simulink model "SiemensBike"  (R2025b)
settings: Solver=ode14x  StartTime=0  StopTime=inf  FixedStep=.01  RelTol=1e-2  EnableMultiTasking=on
StopFcn:
  | %toc
undefined symbols (not defined in the file): CtrlTcuInitGear, EnvAbsPrs, EnvAirTemp, EnvNomFrictionScaling, EnvNominalGrade, EnvWindVelX, EnvWindVelY, EnvWindVelZ, MotoFrmLngth, Sim3dSensor
libraries: vehdynlibviscommon x3, sim3dgroundtruthsensorlib x2, simulink x1, sharedtransform x1, autolibutils x1
(part 2 of 3)

== system SiemensBike/Environment/Friction/Varying Friction ==
  MotoFdbk : Inport
  Bus Selector1 : BusSelector  OutputSignals=Whl.Genrl.Frnt.Cp.Disp.x,Whl.Genrl.Rear.Cp.Disp.x,Whl.Genrl.Frnt.Cp.Disp.y,Whl.Genrl.Rear.Cp.Disp.y
  Bus Selector2 : BusSelector  OutputSignals=Body.InertFrm.Cg.Disp
  Road Track Friction : Subsystem  mask(Road Track Friction){surface_popup=Split friction coefficient scaling factor, lambda_g=EnvNomFrictionScaling, lambda_r=.6, r_x0=175, r_y0=-100, r_xw=1000, r_yw=500, aMode=2}
      mask prompts: surface_popup "vdynblks:vehdynManFriction:blkPrm_surface_popup"; lambda_g "vdynblks:vehdynManFriction:blkPrm_lambda_g"; lambda_r "vdynblks:vehdynManFriction:blkPrm_lambda_r"; r_x0 "vdynblks:vehdynManFriction:blkPrm_r_x0"; r_y0 "vdynblks:vehdynManFriction:blkPrm_r_y0"; r_xw "vdynblks:vehdynManFriction:blkPrm_r_xw"; r_yw "vdynblks:vehdynManFriction:blkPrm_r_yw"
      mask init:
      | % Scaling factor for the friction coefficient around the rectangular region
      | mutable = [lambda_g, lambda_g, lambda_g, lambda_g;
      |            lambda_g, lambda_r, lambda_r, lambda_g; 
      |            lambda_g, lambda_r, lambda_r, lambda_g; 
      |            lambda_g, lambda_g, lambda_g, lambda_g ];
      |        
      | 
      | % The step is distance between breakpoint near the boundary of high and
      | % low friction coefficient
      | 
      | step = 0.01 ; 
      | 
      | % In the mask initialization, xbr and ybr breakpoints are with respect to
      | % Body fixed coordinate system. At time t=0, xbr and ybr breakpoints
      | % updates to Earth (Inertial) Fixed coordinate system. The breakpoints for
      | % the lookup table are added via inputs.
      | 
      | xbr = [(r_x0 - step) , (r_x0 + step), (r_x0 + r_xw - step) , (r_x0 + r_xw + step) ];
      | ybr = [(r_y0 - step) , (r_y0 + step), (r_y0 + r_yw - step) , (r_y0 + r_yw + step) ];
      | 
      | 
      | % To check if the created track is split mu or constant mu
      | 
      | surface_popup = get_param(gcb, 'surface_popup');
      | 
      | if strcmp(surface_popup, 'Split friction coefficient scaling factor')
      |     SplitLambdaTrck = 1;
      | elseif strcmp(surface_popup, 'Constant friction coefficient scaling factor')
      |     SplitLambdaTrck = 0;
      | end
      mask Help: eval('vdynblkshelp(''vdynblkstrack'')');
      mask TypeOptions surface_popup: vdynblks:vehdynManFriction:blkCmb_surface_popup_c1 | vdynblks:vehdynManFriction:blkCmb_surface_popup_c2
      mask Callback surface_popup:
      | surface_popup = get_param(gcb, 'surface_popup');
      | m = Simulink.Mask.get(gcb);
      | 
      | lambda_g = m.getParameter('lambda_g');
      | lambda_r = m.getParameter('lambda_r');
      | r_x0 = m.getParameter('r_x0');
      | r_y0 = m.getParameter('r_y0');
      | r_xw = m.getParameter('r_xw');
      | r_yw = m.getParameter('r_yw');
      | %track_view = m.getParameter('track_view');
      | 
      | 
      | if strcmp(surface_popup, 'Split friction coefficient scaling factor')
      |     lambda_g.Visible = 'on';
      |     lambda_r.Visible = 'on';
      |     r_x0.Visible = 'on';
      |     r_y0.Visible = 'on';
      |     r_xw.Visible = 'on';
      |     r_yw.Visible = 'on';
      |     %track_view.Visible = 'on';
      | 
      | elseif strcmp(surface_popup,'Constant friction coefficient scaling factor')
      |     lambda_g.Visible = 'on';
      |     lambda_r.Visible = 'off';
      |     r_x0.Visible = 'off';
      |     r_y0.Visible = 'off';
      |     r_xw.Visible = 'off';
      |     r_yw.Visible = 'off';
      |     %track_view.Visible = 'off';
      | end
      | [~]=autosharedicon('autolibutils',gcb,0);
      mask DialogControl DescGroupVar Prompt: Road Track Friction
      mask DialogControl DescTextVar Prompt: vdynblks:vehdynManFriction:blkDesc
      mask DialogControl surface_popup Prompt: Type of surface:
      mask DialogControl lambda_g Prompt: Scaling factor for the friction coefficient of ground, lambda_g :
      mask DialogControl lambda_r Prompt: Scaling factor for the friction coefficient of rectangular surface, lambda_r :
      mask DialogControl r_x0 Prompt: X coordinate of lower left corner of rectangular surface, r_x0 [m]:
      mask DialogControl r_y0 Prompt: Y coordinate of lower left corner of rectangular surface, r_y0 [m]:
      mask DialogControl r_xw Prompt: Rectangular surface width in X direction, r_xw [m]:
      mask DialogControl r_yw Prompt: Rectangular surface width in Y direction, r_yw [m]:
  Wheel Coordinates : Subsystem
  FricCoeffLambda : Outport
  wires:
  Wheel Coordinates/1(XWhl) -> Road Track Friction/1(XWhl)
  MotoFdbk/1 -> Bus Selector2/1, Bus Selector1/1
  Wheel Coordinates/2(YWhl) -> Road Track Friction/2(YWhl)
  Road Track Friction/1(FricCoeffLambda) -> FricCoeffLambda/1
  Bus Selector2/1 -> Road Track Friction/3(Cg)  "<Disp>"
  Bus Selector1/1 -> Wheel Coordinates/1(FrntAxlX)  "<x>"
  Bus Selector1/2 -> Wheel Coordinates/2(RearAxlX)  "<x>"
  Bus Selector1/3 -> Wheel Coordinates/3(FrntAxlY)  "<y>"
  Bus Selector1/4 -> Wheel Coordinates/4(RearAxlY)  "<y>"

== system SiemensBike/Environment/Ground Feedback/3D Engine ==
  Friction : Inport
  WheelFdbk : Inport  Port=2
  3D Engine Source : Subsystem  Variant=on  VariantControl=Choice  mask(Terrain Source){terrType=Single point}
      mask prompts: terrType "Terrain feedback type:"
      mask help:
      | This variant subsystem provides the option for:
      | - a single point of contact for each wheel with minimal post-processing ideal for smooth surfaces and maximum run-time performance.
      | - multiple points of contact per wheel which may be used when interested in non-smooth terrain at a higher computational cost and requires Vehicle Dynamics Blockset.
      mask TypeOptions terrType: Single point | Multiple points
  Bus Creator2 : BusCreator  Inputs=2
  Bus Creator3 : BusCreator  Inputs=3
  Demux1 : Demux  Outputs=2
  Signal Specification1 : SignalSpecification  Unit=1
  Ground : Outport  VectorParamsAs1DForOutWhenUnconnected=off
  wires:
  3D Engine Source/2(DCM) -> Bus Creator3/2  "DCM"
  3D Engine Source/1(z) -> Bus Creator3/1  "z"
  WheelFdbk/1 -> 3D Engine Source/1(WheelFdbk)
  Friction/1 -> Signal Specification1/1
  Bus Creator3/1 -> Ground/1
  Bus Creator2/1 -> Bus Creator3/3  "mu"
  Demux1/2 -> Bus Creator2/2  "mu_R"
  Demux1/1 -> Bus Creator2/1  "mu_F"
  Signal Specification1/1 -> Demux1/1

== system SiemensBike/Environment/Ground Feedback/Constant ==
  Friction : Inport
  Bus Creator : BusCreator  Inputs=2
  Bus Creator2 : BusCreator  Inputs=2
  Bus Creator3 : BusCreator  Inputs=3
  Constant1 : Constant  Value=zeros(2,1)
  Constant2 : Constant  Value=repmat(eye(3),1,1,2)  SampleTime=-1
  Demux : Demux  Outputs=2
  Demux1 : Demux  Outputs=2
  Signal Specification : SignalSpecification  Unit=m
  Signal Specification1 : SignalSpecification  Unit=1
  Ground : Outport  VectorParamsAs1DForOutWhenUnconnected=off
  wires:
  Constant1/1 -> Signal Specification/1
  Signal Specification/1 -> Demux/1
  Demux/1 -> Bus Creator/1  "G_F_z"
  Demux/2 -> Bus Creator/2  "G_R_z"
  Bus Creator/1 -> Bus Creator3/1  "z"
  Demux1/1 -> Bus Creator2/1  "mu_F"
  Demux1/2 -> Bus Creator2/2  "mu_R"
  Bus Creator2/1 -> Bus Creator3/3  "mu"
  Friction/1 -> Signal Specification1/1
  Signal Specification1/1 -> Demux1/1
  Bus Creator3/1 -> Ground/1
  Constant2/1 -> Bus Creator3/2  "DCM"

== system SiemensBike/Motorcycle Vehicle/Body, Steer, Suspension, Wheels/Body, Steer, Suspension, Wheels ==
  WindXYZ : Inport
  BrkPrs : Inport  Port=2
  MDrvSprtR : Inport  Port=3
  MDrvArmR : Inport  Port=4
  MDrvFrm : Inport  Port=5
  ScaleFactrs : Inport  Port=6
  SteerCmd : Inport  Port=7
  In_Plane_Model : Subsystem  VariantControl=In_Plane_Model  ReferencedSubsystem=In_Plane_Model
  Out_of_Plane_Model : Subsystem  VariantControl=Out_of_Plane_Model  ReferencedSubsystem=Out_of_Plane_Model
  Moto : Outport
  Wheels : Outport  Port=2

== system SiemensBike/Motorcycle Vehicle/Body, Steer, Suspension, Wheels/Chassis Input ==
  Env : Inport
  Driveline : Inport  Port=2
  Rider : Inport  Port=3
  Bus Selector : BusSelector  OutputSignals=SteerFdbk
  Bus Selector2 : BusSelector  OutputSignals=Wind,Gnd.mu
  Bus Selector4 : BusSelector  OutputSignals=BrkPrs,Info.ChainInfo.MDrvSprtR,Info.MDrvArmR,Info.MDrvFrm
  Bus to Vector : BusToVector
  Wind : Outport  VectorParamsAs1DForOutWhenUnconnected=off
  BrkPrs : Outport  Port=2  VectorParamsAs1DForOutWhenUnconnected=off
  MDrvSprtR : Outport  Port=3  VectorParamsAs1DForOutWhenUnconnected=off
  MDrvArmR : Outport  Port=4  VectorParamsAs1DForOutWhenUnconnected=off
  MDrvFrm : Outport  Port=5  VectorParamsAs1DForOutWhenUnconnected=off
  ScaleFactrs : Outport  Port=6  VectorParamsAs1DForOutWhenUnconnected=off
  SteerCmd : Outport  Port=7  VectorParamsAs1DForOutWhenUnconnected=off
  wires:
  Env/1 -> Bus Selector2/1
  Bus Selector2/1 -> Wind/1  "<Wind>"
  Driveline/1 -> Bus Selector4/1
  Bus Selector4/4 -> MDrvFrm/1  "<MDrvFrm>"
  Bus Selector4/3 -> MDrvArmR/1  "<MDrvArmR>"
  Bus Selector4/2 -> MDrvSprtR/1  "<MDrvSprtR>"
  Bus Selector4/1 -> BrkPrs/1  "<BrkPrs>"
  Bus Selector2/2 -> Bus to Vector/1  "<mu>"
  Bus to Vector/1 -> ScaleFactrs/1
  Rider/1 -> Bus Selector/1
  Bus Selector/1 -> SteerCmd/1  "<SteerFdbk>"

== system SiemensBike/Motorcycle Vehicle/Body, Steer, Suspension, Wheels/Chassis Output ==
  Moto : Inport
  Wheels : Inport  Port=2
  Out Bus Element4 : Outport  PortName=MotoFdbk
  Out Bus Element1 : Outport  Port=2  PortName=WheelsFdbk
  wires:
  Moto/1 -> Out Bus Element4/1
  Wheels/1 -> Out Bus Element1/1

== system SiemensBike/Motorcycle Vehicle/Control Feedback/Variant Subsystem ==
  note: 1) Add Subsystem or Model blocks as valid variant choices.
      | 2) You cannot connect blocks at this level. At simulation, connectivity is automatically
      | determined, based on the active variant and port name matching.
  MotoFdbk : Inport
  IMU_Sensor : Subsystem  VariantControl=IMU_Sensor  ReferencedSubsystem=IMU_Sensor
  No_IMU_Sensor : Subsystem  VariantControl=No_IMU_Sensor  ReferencedSubsystem=No_IMU_Sensor
  IMU : Outport

== system SiemensBike/Motorcycle Vehicle/Hand Levers and Pedals/Hand Levers and Pedals ==
  note: Placeholder for introducing faults, detailed actuator behavior,
      | interactions of other systems with a human interface such
      | as changes in power steering and braking assistance.
  SteerCmd : Inport
  AccCmd : Inport  Port=2
  DecelCmd : Inport  Port=3
  GearCmd : Inport  Port=4
  BrkPrs : Inport  Port=5
  StrWhlTrq : Inport  Port=6
  Brake Pedal : Subsystem
  Dead Zone3 : DeadZone  LowerValue=-.01  UpperValue=.01  ZeroCross=off
  Terminator : Terminator
  Terminator1 : Terminator
  Twist2Acc : Lookup_n-D  NumberOfTableDimensions=1  BreakpointsForDimension1=[0 1]  Table=[0 1]  ExtrapMethod=Clip  InternalRulePriority=Speed  RndMeth=Simplest
  SteerFdbk : Outport
  AccFdbk : Outport  Port=2
  DecelFdbk : Outport  Port=3
  GearFdbk : Outport  Port=4
  wires:
  SteerCmd/1 -> Dead Zone3/1
  DecelCmd/1 -> Brake Pedal/1(DecelCmd)
  GearCmd/1 -> GearFdbk/1
  BrkPrs/1 -> Terminator/1
  StrWhlTrq/1 -> Terminator1/1
  Brake Pedal/1(DecelFdbk) -> DecelFdbk/1
  Dead Zone3/1 -> SteerFdbk/1
  AccCmd/1 -> Twist2Acc/1
  Twist2Acc/1 -> AccFdbk/1

== system SiemensBike/Motorcycle Vehicle/Hand Levers and Pedals/Pedal Cluster Input ==
  Rider : Inport
  Driveline : Inport  Port=2
  Bus Selector : BusSelector  OutputSignals=SteerCmd,AccelCmd,DecelCmd,GearCmd
  Bus Selector1 : BusSelector  OutputSignals=EMSpd
  Constant : Constant  Value=0
  SteerCmd : Outport  VectorParamsAs1DForOutWhenUnconnected=off
  AccelCmd : Outport  Port=2  VectorParamsAs1DForOutWhenUnconnected=off
  DecelCmd : Outport  Port=3  VectorParamsAs1DForOutWhenUnconnected=off
  GearCmd : Outport  Port=4  VectorParamsAs1DForOutWhenUnconnected=off
  BrkPrs : Outport  Port=5  VectorParamsAs1DForOutWhenUnconnected=off
  StrWhlTrq : Outport  Port=6  VectorParamsAs1DForOutWhenUnconnected=off
  wires:
  Bus Selector/2 -> AccelCmd/1  "<AccelCmd>"
  Rider/1 -> Bus Selector/1
  Bus Selector/3 -> DecelCmd/1  "<DecelCmd>"
  Bus Selector/4 -> GearCmd/1  "<GearCmd>"
  Bus Selector/1 -> SteerCmd/1  "<SteerCmd>"
  Driveline/1 -> Bus Selector1/1
  Bus Selector1/1 -> BrkPrs/1  "<EMSpd>"
  Constant/1 -> StrWhlTrq/1

== system SiemensBike/Motorcycle Vehicle/Hand Levers and Pedals/Pedal Cluster Output ==
  SteerFdbk : Inport
  AccFdbk : Inport  Port=2
  DecelFdbk : Inport  Port=3
  GearFdbk : Inport  Port=4
  Bus Creator1 : BusCreator  Inputs=4
  Signal Specification : SignalSpecification  Unit=N*m
  Signal Specification1 : SignalSpecification  Unit=1
  Signal Specification2 : SignalSpecification  Unit=1
  Signal Specification3 : SignalSpecification  Unit=1
  OperatorFdbk : Outport
  wires:
  Signal Specification1/1 -> Bus Creator1/2  "AccFdbk"
  Signal Specification3/1 -> Bus Creator1/4  "GearFdbk"
  AccFdbk/1 -> Signal Specification1/1
  DecelFdbk/1 -> Signal Specification2/1
  GearFdbk/1 -> Signal Specification3/1
  Signal Specification/1 -> Bus Creator1/1  "SteerFdbk"
  SteerFdbk/1 -> Signal Specification/1
  Bus Creator1/1 -> OperatorFdbk/1
  Signal Specification2/1 -> Bus Creator1/3  "DecelFdbk"

== system SiemensBike/Motorcycle Vehicle/Propulsion System/Actuators ==
  note: 1) Add Subsystem or Model blocks as valid variant choices.
      | 2) You cannot connect blocks at this level. At simulation, connectivity is automatically
      | determined, based on the active variant and port name matching.
  TrqCmd : Inport
  EngSpd : Inport  Port=2
  EMTrqCmd : Inport  Port=3
  EMSpd : Inport  Port=4
  AmbTemp : Inport  Port=5
  MotoElectricalSystem : Subsystem  VariantControl=MotoElectricalSystem  ReferencedSubsystem=MotoElectricalSystem
  MotoMappedEngine : Subsystem  VariantControl=MotoMappedEngine  ReferencedSubsystem=MotoMappedEngine
  MotoSimpleEngine : Subsystem  VariantControl=MotoSimpleEngine  ReferencedSubsystem=MotoSimpleEngine
  Eng : Outport
  Battery : Outport  Port=2
  ElecMachine : Outport  Port=3

== system SiemensBike/Motorcycle Vehicle/Propulsion System/Electrical System Input ==
  Cntrl : Inport
  Driveline : Inport  Port=2
  Env : Inport  Port=3
  Bus Selector : BusSelector  OutputSignals=VCU.EMTrqCmd
  Bus Selector1 : BusSelector  OutputSignals=EMSpd
  Bus Selector2 : BusSelector  OutputSignals=Temp
  First Order Hold : FirstOrderHold  ErrorTolerance=inf  AllowContinuousInput=on
  EMTrqCmd : Outport  VectorParamsAs1DForOutWhenUnconnected=off
  EMSpd : Outport  Port=2  VectorParamsAs1DForOutWhenUnconnected=off
  AmbTemp : Outport  Port=3  VectorParamsAs1DForOutWhenUnconnected=off
  wires:
  Cntrl/1 -> Bus Selector/1
  Bus Selector/1 -> First Order Hold/1  "<EMTrqCmd>"
  Bus Selector1/1 -> EMSpd/1  "<EMSpd>"
  Env/1 -> Bus Selector2/1
  Bus Selector2/1 -> AmbTemp/1  "<Temp>"
  Driveline/1 -> Bus Selector1/1
  First Order Hold/1 -> EMTrqCmd/1

== system SiemensBike/Motorcycle Vehicle/Propulsion System/Engine Input ==
  Cntrl : Inport
  Driveline : Inport  Port=2
  Bus Selector : BusSelector  OutputSignals=ECU.EngTrqCmd
  Bus Selector1 : BusSelector  OutputSignals=EngSpd
  First Order Hold : FirstOrderHold  OutputAlgorithm=Fast (Minimize Error)  ErrorTolerance=.01  AllowContinuousInput=on
  EngTrqCmd : Outport  VectorParamsAs1DForOutWhenUnconnected=off
  EngSpd : Outport  Port=2  VectorParamsAs1DForOutWhenUnconnected=off
  wires:
  Driveline/1 -> Bus Selector1/1
  Cntrl/1 -> Bus Selector/1
  Bus Selector/1 -> First Order Hold/1  "<EngTrqCmd>"
  Bus Selector1/1 -> EngSpd/1  "<EngSpd>"
  First Order Hold/1 -> EngTrqCmd/1

== system SiemensBike/Motorcycle Vehicle/Transmission, Driveline and Brakes/Brake Hydraulics ==
  BrkPrsCmd : Inport
  Front Bias : Constant
  Gain4 : Gain  Gain=8e6
  Mux : Mux  Inputs=2
  Product : Product
  Rear Bias : Constant  Value=.6
  Valve : autolibutils/Cont LPF  wc=20*2*pi  AbsoluteTolerance=auto  aMode=2
  BrkPrs : Outport  VectorParamsAs1DForOutWhenUnconnected=off
  wires:
  Valve/1 -> Product/2
  Gain4/1 -> BrkPrs/1
  BrkPrsCmd/1 -> Valve/1
  Front Bias/1 -> Mux/1
  Rear Bias/1 -> Mux/2
  Product/1 -> Gain4/1
  Mux/1 -> Product/1

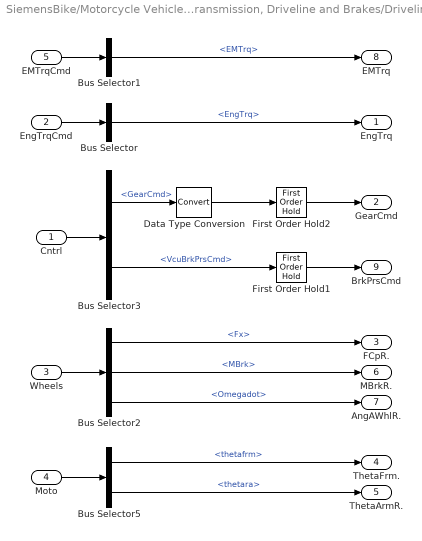
== system SiemensBike/Motorcycle Vehicle/Transmission, Driveline and Brakes/Driveline Input ==
  Cntrl : Inport
  EngTrqCmd : Inport  Port=2
  Wheels : Inport  Port=3
  Moto : Inport  Port=4
  EMTrqCmd : Inport  Port=5
  Bus Selector : BusSelector  OutputSignals=EngTrq
  Bus Selector1 : BusSelector  OutputSignals=EMTrq
  Bus Selector2 : BusSelector  OutputSignals=RearTire.Fx,RearTire.MBrk,RearTire.Omegadot
  Bus Selector3 : BusSelector  OutputSignals=Transmission.GearCmd,VCU.VcuBrkPrsCmd
  Bus Selector5 : BusSelector  OutputSignals=Frame.Genrl.Ang.thetafrm,RearArm.Genrl.Ang.thetara
  Data Type Conversion : DataTypeConversion  SaturateOnIntegerOverflow=off  RndMeth=Floor
  First Order Hold1 : FirstOrderHold  OutputAlgorithm=Fast (Minimize Error)  ErrorTolerance=.001  AllowContinuousInput=on
  First Order Hold2 : FirstOrderHold  InitialOutput=CtrlTcuInitGear  ErrorTolerance=.5  AllowContinuousInput=on
  EngTrq : Outport  VectorParamsAs1DForOutWhenUnconnected=off
  GearCmd : Outport  Port=2  VectorParamsAs1DForOutWhenUnconnected=off
  FCpR. : Outport  Port=3  VectorParamsAs1DForOutWhenUnconnected=off
  ThetaFrm. : Outport  Port=4  VectorParamsAs1DForOutWhenUnconnected=off
  ThetaArmR. : Outport  Port=5  VectorParamsAs1DForOutWhenUnconnected=off
  MBrkR. : Outport  Port=6  VectorParamsAs1DForOutWhenUnconnected=off
  AngAWhlR. : Outport  Port=7  VectorParamsAs1DForOutWhenUnconnected=off
  EMTrq : Outport  Port=8  VectorParamsAs1DForOutWhenUnconnected=off
  BrkPrsCmd : Outport  Port=9  VectorParamsAs1DForOutWhenUnconnected=off
  wires:
  Wheels/1 -> Bus Selector2/1
  Moto/1 -> Bus Selector5/1
  Bus Selector2/3 -> AngAWhlR./1  "<Omegadot>"
  Bus Selector2/2 -> MBrkR./1  "<MBrk>"
  Bus Selector2/1 -> FCpR./1  "<Fx>"
  Bus Selector5/2 -> ThetaArmR./1  "<thetara>"
  Bus Selector5/1 -> ThetaFrm./1  "<thetafrm>"
  EngTrqCmd/1 -> Bus Selector/1
  EMTrqCmd/1 -> Bus Selector1/1
  Bus Selector3/2 -> First Order Hold1/1  "<VcuBrkPrsCmd>"
  Bus Selector3/1 -> Data Type Conversion/1  "<GearCmd>"
  Cntrl/1 -> Bus Selector3/1
  Bus Selector/1 -> EngTrq/1  "<EngTrq>"
  Bus Selector1/1 -> EMTrq/1  "<EMTrq>"
  First Order Hold1/1 -> BrkPrsCmd/1
  Data Type Conversion/1 -> First Order Hold2/1
  First Order Hold2/1 -> GearCmd/1

== system SiemensBike/Motorcycle Vehicle/Transmission, Driveline and Brakes/Driveline Output ==
  EngSpd : Inport
  Gear : Inport  Port=2
  Info : Inport  Port=3
  EMSpd : Inport  Port=4
  BrkPrs : Inport  Port=5
  Bus Creator1 : BusCreator  Inputs=7
  Ground{,1..3} (4 alike) : Ground
  Mux : Mux  Inputs=2
  Mux1 : Mux  Inputs=2
  Signal Specification7 : SignalSpecification  Unit=Pa  Dimensions=2
  Driveline : Outport  VectorParamsAs1DForOutWhenUnconnected=off
  wires:
  Bus Creator1/1 -> Driveline/1  "Driveline"
  EngSpd/1 -> Bus Creator1/3  "EngSpd"
  EMSpd/1 -> Bus Creator1/2  "EMSpd"
  Gear/1 -> Bus Creator1/4  "Gear"
  Info/1 -> Bus Creator1/7  "Info"
  Mux/1 -> Bus Creator1/6  "AxlTrq"
  Mux1/1 -> Bus Creator1/5  "PropShftSpd"
  Ground3/1 -> Mux/2
  Ground2/1 -> Mux/1
  Ground/1 -> Mux1/1
  Ground1/1 -> Mux1/2
  BrkPrs/1 -> Signal Specification7/1
  Signal Specification7/1 -> Bus Creator1/1  "BrkPrs"

== system SiemensBike/Motorcycle Vehicle/Transmission, Driveline and Brakes/Transmission and Driveline ==
  EngTrq : Inport
  GearCmd : Inport  Port=2
  FCpR : Inport  Port=3
  ThetaFrm : Inport  Port=4
  ThetaArmR : Inport  Port=5
  MBrkR : Inport  Port=6
  AngAWhlR : Inport  Port=7
  EMTrq : Inport  Port=8
  Driveline : Subsystem  Variant=on  VariantChoicesSpecifier={'Chain_Drive', 'No_Chain_Drive'}  VariantControlMode=label  VariantControl=Choice  LabelModeActiveChoice=Chain_Drive
  Transmission : Subsystem  Variant=on  VariantChoicesSpecifier={'ConventionalMotorcycle', 'ElectricMotorcycle'}  VariantControlMode=label  VariantControl=Choice  LabelModeActiveChoice=ConventionalMotorcycle
  EngSpd : Outport
  Gear : Outport  Port=2
  Info : Outport  Port=3
  EMSpd : Outport  Port=4
  wires:
  EngTrq/1 -> Transmission/1(EngTrq)
  GearCmd/1 -> Transmission/2(GearCmd)
  FCpR/1 -> Driveline/1(FCpR)
  ThetaFrm/1 -> Driveline/2(ThetaFrm)
  ThetaArmR/1 -> Driveline/3(ThetaArmR)
  MBrkR/1 -> Driveline/4(MBrkR)
  AngAWhlR/1 -> Driveline/5(AngAWhlR)
  EMTrq/1 -> Transmission/3(EMTrq)
  Driveline/2(DrvSprktSpd) -> Transmission/4(DrvSprktSpd)
  Transmission/4(DrvSprktTrq) -> Driveline/6(DrvSprktTrq)
  Driveline/1(Info) -> Info/1
  Transmission/1(EngSpd) -> EngSpd/1
  Transmission/2(Gear) -> Gear/1
  Transmission/3(EMSpd) -> EMSpd/1

== system SiemensBike/Visualization/ISO 15037-1:2006/Disabled ==
  VehFdbk : Inport
  Terminator1 : Terminator
  wires:
  VehFdbk/1 -> Terminator1/1

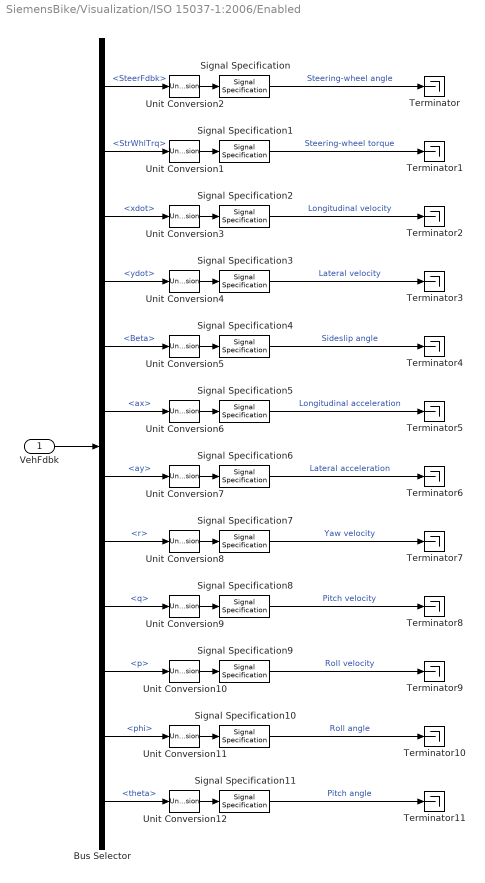
== system SiemensBike/Visualization/ISO 15037-1:2006/Enabled ==
  VehFdbk : Inport
  Bus Selector : BusSelector  OutputSignals=Rider.SteerFdbk,Steering.StrWhlTrq,Body.BdyFrm.Cg.Vel.xdot,Body.BdyFrm.Cg.Vel.ydot,Body.BdyFrm.Cg.Ang.Beta,Body.BdyFrm.Cg.Acc.ax,Body.BdyFrm.Cg.Acc.ay,Body.BdyFrm.Cg.AngVel.r,Body.BdyFrm.Cg.AngVel.q,Body.BdyFrm.Cg.AngVel.p,Body.InertFrm.Cg.Ang.phi,Body.InertFrm.Cg.Ang.theta
  Signal Specification{,4,10..11} (4 alike) : SignalSpecification  Unit=deg
  Signal Specification1 : SignalSpecification  Unit=N*m
  Signal Specification2 : SignalSpecification  Unit=km/h
  Signal Specification3 : SignalSpecification  Unit=m/s
  Signal Specification5 : SignalSpecification  Unit=m/s^2
  Signal Specification6 : SignalSpecification  Unit=m/s^2
  Signal Specification7 : SignalSpecification  Unit=deg/s
  Signal Specification8 : SignalSpecification  Unit=deg/s
  Signal Specification9 : SignalSpecification  Unit=deg/s
  Terminator{,1..11} (12 alike) : Terminator
  Unit Conversion{1..12} (12 alike) : UnitConversion
  wires:
  Bus Selector/12 -> Unit Conversion12/1  "<theta>"
  Signal Specification11/1 -> Terminator11/1  "Pitch angle"
  Unit Conversion12/1 -> Signal Specification11/1
  Bus Selector/11 -> Unit Conversion11/1  "<phi>"
  Unit Conversion11/1 -> Signal Specification10/1
  Signal Specification10/1 -> Terminator10/1  "Roll angle"
  Bus Selector/10 -> Unit Conversion10/1  "<p>"
  Signal Specification9/1 -> Terminator9/1  "Roll velocity"
  Unit Conversion10/1 -> Signal Specification9/1
  Bus Selector/9 -> Unit Conversion9/1  "<q>"
  Unit Conversion9/1 -> Signal Specification8/1
  Signal Specification8/1 -> Terminator8/1  "Pitch velocity"
  Bus Selector/8 -> Unit Conversion8/1  "<r>"
  Signal Specification7/1 -> Terminator7/1  "Yaw velocity"
  Unit Conversion8/1 -> Signal Specification7/1
  Bus Selector/7 -> Unit Conversion7/1  "<ay>"
  Unit Conversion7/1 -> Signal Specification6/1
  Signal Specification6/1 -> Terminator6/1  "Lateral acceleration"
  Bus Selector/6 -> Unit Conversion6/1  "<ax>"
  Signal Specification5/1 -> Terminator5/1  "Longitudinal acceleration"
  Unit Conversion6/1 -> Signal Specification5/1
  Bus Selector/5 -> Unit Conversion5/1  "<Beta>"
  Unit Conversion5/1 -> Signal Specification4/1
  Signal Specification4/1 -> Terminator4/1  "Sideslip angle"
  Bus Selector/4 -> Unit Conversion4/1  "<ydot>"
  Signal Specification3/1 -> Terminator3/1  "Lateral velocity"
  Unit Conversion4/1 -> Signal Specification3/1
  Bus Selector/3 -> Unit Conversion3/1  "<xdot>"
  Unit Conversion3/1 -> Signal Specification2/1
  Signal Specification2/1 -> Terminator2/1  "Longitudinal velocity"
  Signal Specification1/1 -> Terminator1/1  "Steering-wheel torque"
  Unit Conversion1/1 -> Signal Specification1/1
  Bus Selector/2 -> Unit Conversion1/1  "<StrWhlTrq>"
  Signal Specification/1 -> Terminator/1  "Steering-wheel angle"
  Unit Conversion2/1 -> Signal Specification/1
  VehFdbk/1 -> Bus Selector/1
  Bus Selector/1 -> Unit Conversion2/1  "<SteerFdbk>"

== system SiemensBike/Visualization/Scope Type/DLC ==
  VehFdbk : Inport
  Vis : Inport  Port=2
  Bus Creator : BusCreator  Inputs=3
  Bus Selector3 : BusSelector  OutputSignals=Body.InertFrm.Cg.Disp.X,Body.InertFrm.Cg.Disp.Z
  Bus Selector4 : BusSelector  OutputSignals=LeftBnd,RightBnd,LtrlRef
  Lane Change : Scope
      settings: Title=Double Lane Change: Lateral Displacement  ActiveDisplayYMinimum=-3.28469  ActiveDisplayYMaximum=6.06905  YLabel=Lateral Displacement [m] (positive = right direction)  DataLoggingSaveFormat=Array
  Mux1 : Mux  Inputs=3
  Rate Transition : RateTransition  OutPortSampleTime=.1
  Rate Transition3 : RateTransition  OutPortSampleTime=.1
  Signal Copy : SignalConversion  OverrideOpt=off
  Signal Copy1 : SignalConversion  OverrideOpt=off
  Signal Copy2 : SignalConversion  OverrideOpt=off
  Ref : Outport  VectorParamsAs1DForOutWhenUnconnected=off
  wires:
  VehFdbk/1 -> Bus Selector3/1
  Vis/1 -> Bus Selector4/1
  Bus Creator/1 -> Ref/1
  Bus Selector3/2 -> Signal Copy2/1  "<Z>"
  Signal Copy/1 -> Bus Creator/2  "YRef"
  Signal Copy1/1 -> Bus Creator/1  "XRef"
  Signal Copy2/1 -> Bus Creator/3  "ZRef"
  Rate Transition3/1 -> Mux1/2  "Right Boundary"
  Bus Selector4/3 -> Signal Copy/1, Mux1/3  "<LtrlRef>"
  Mux1/1 -> Lane Change/1
  Bus Selector4/1 -> Rate Transition/1  "<LeftBnd>"
  Rate Transition/1 -> Mux1/1  "Left Boundary"
  Bus Selector4/2 -> Rate Transition3/1  "<RightBnd>"
  Bus Selector3/1 -> Signal Copy1/1  "<X>"

== system SiemensBike/Visualization/Scope Type/None ==
  VehFdbk : Inport
  Vis : Inport  Port=2
  Bus Selector2 : BusSelector  OutputSignals=Steer.Genrl.Ang.thetasteer
  Bus Selector9 : BusSelector  OutputSignals=Body.BdyFrm.Cg.AngVel.r
  Signal Specification3 : SignalSpecification  Unit=deg/s
  Unit Conversion4 : UnitConversion
  Yaw Rate and Steer : Scope  NumInputPorts=2
      settings: ActiveDisplayYMinimum=-112.49987  ActiveDisplayYMaximum=112.49996
  Ref : Outport  VectorParamsAs1DForOutWhenUnconnected=off
  wires:
  Bus Selector9/1 -> Unit Conversion4/1  "<r>"
  Signal Specification3/1 -> Yaw Rate and Steer/1
  Unit Conversion4/1 -> Signal Specification3/1
  VehFdbk/1 -> Bus Selector2/1, Bus Selector9/1  "VehFdbk"
  Bus Selector2/1 -> Yaw Rate and Steer/2  "<thetasteer>"
  Vis/1 -> Ref/1

== system SiemensBike/Visualization/Scope Type/XYZ ==
  VehFdbk : Inport
  Vis : Inport  Port=2
  Terminator : Terminator
  Ref : Outport  VectorParamsAs1DForOutWhenUnconnected=off
  wires:
  Vis/1 -> Ref/1
  VehFdbk/1 -> Terminator/1

== system SiemensBike/Visualization/Vehicle XY Plotter/Disabled ==

== system SiemensBike/Visualization/Vehicle XY Plotter/XY View ==
  Bus Element In2 : Inport  PortName=VehFdbk
  Bus Selector1 : BusSelector  OutputSignals=Body.InertFrm.Cg.Ang.phi,Body.InertFrm.Cg.Ang.theta,Body.InertFrm.Cg.Ang.psi  OutputAsBus=on
  Bus Selector2 : BusSelector  OutputSignals=Wheels.FrontTire.Fx,Wheels.RearTire.Fx
  Bus Selector3 : BusSelector  OutputSignals=Wheels.FrontTire.Fy,Wheels.RearTire.Fy
  Bus Selector5 : BusSelector  OutputSignals=Wheels.FrontTire.Alpha,Wheels.RearTire.Alpha
  Bus Selector6 : BusSelector  OutputSignals=Body.InertFrm.Cg.Disp.X,Body.InertFrm.Cg.Disp.Y,Body.InertFrm.Cg.Disp.Z  OutputAsBus=on
  Bus Selector7 : BusSelector  OutputSignals=Body.InertFrm.Cg.Vel.Xdot,Body.InertFrm.Cg.Vel.Ydot,Body.InertFrm.Cg.Vel.Zdot  OutputAsBus=on
  Bus Selector9 : BusSelector  OutputSignals=Driveline.EngSpd,Driveline.EMSpd,Driveline.Gear
  Bus to Vector : BusToVector
  Bus to Vector1 : BusToVector
  Bus to Vector2 : BusToVector
  Max : MinMax  Function=max  Inputs=2
  Multi-Track XY Plotter : vehdynlibviscommon/Multi-Track XY Plotter  numTrack=Single track  extRef=off  extStats=on  extTireF=on  a=1.5  b=1.5  w=0  figBorder=10  bufferSize=1024  velNorm=5  tireFNorm=1000  pltDT=.1
      settings: LibrarySourceBlock=vehdynlibviscommon/Vehicle XY Plot Configuration
  Mux{,1..3} (4 alike) : Mux  Inputs=2
  Unary Minus : UnaryMinus
  wires:
  Bus Selector7/1 -> Bus to Vector1/1
  Bus to Vector1/1 -> Multi-Track XY Plotter/3
  Bus Selector2/1 -> Mux1/1  "<Fx>"
  Bus Selector1/1 -> Bus to Vector2/1
  Bus Selector9/1 -> Max/1  "<EngSpd>"
  Bus to Vector/1 -> Multi-Track XY Plotter/1
  Bus Selector6/1 -> Bus to Vector/1
  Bus to Vector2/1 -> Multi-Track XY Plotter/2
  Bus Element In2/1 -> Bus Selector3/1, Bus Selector2/1, Bus Selector9/1, Bus Selector5/1, Bus Selector7/1, Bus Selector1/1, Bus Selector6/1  "VehFdbk"
  Mux3/1 -> Multi-Track XY Plotter/4
  Mux1/1 -> Multi-Track XY Plotter/6
  Mux2/1 -> Unary Minus/1
  Max/1 -> Mux/1
  Bus Selector9/2 -> Max/2  "<EMSpd>"
  Mux/1 -> Multi-Track XY Plotter/5
  Bus Selector9/3 -> Mux/2  "<Gear>"
  Bus Selector2/2 -> Mux1/2  "<Fx>"
  Bus Selector3/2 -> Mux2/2  "<Fy>"
  Bus Selector3/1 -> Mux2/1  "<Fy>"
  Bus Selector5/1 -> Mux3/1  "<Alpha>"
  Bus Selector5/2 -> Mux3/2  "<Alpha>"
  Unary Minus/1 -> Multi-Track XY Plotter/7

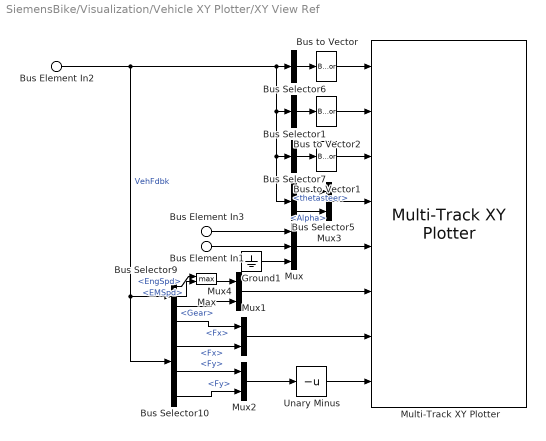
== system SiemensBike/Visualization/Vehicle XY Plotter/XY View Ref ==
  Bus Element In2 : Inport  PortName=VehFdbk
  Bus Element In1 : Inport  Port=2  PortName=Ref  Element=YRef
  Bus Element In3 : Inport  Port=2  PortName=Ref  Element=XRef
  Bus Selector1 : BusSelector  OutputSignals=Body.InertFrm.Cg.Ang.phi,Body.InertFrm.Cg.Ang.theta,Body.InertFrm.Cg.Ang.psi  OutputAsBus=on
  Bus Selector10 : BusSelector  OutputSignals=Wheels.FrontTire.Fx,Wheels.RearTire.Fx,Wheels.FrontTire.Fy,Wheels.RearTire.Fy
  Bus Selector5 : BusSelector  OutputSignals=Steer.Genrl.Ang.thetasteer,Wheels.RearTire.Alpha
  Bus Selector6 : BusSelector  OutputSignals=Body.InertFrm.Cg.Disp.X,Body.InertFrm.Cg.Disp.Y,Body.InertFrm.Cg.Disp.Z  OutputAsBus=on
  Bus Selector7 : BusSelector  OutputSignals=Body.InertFrm.Cg.Vel.Xdot,Body.InertFrm.Cg.Vel.Ydot,Body.InertFrm.Cg.Vel.Zdot  OutputAsBus=on
  Bus Selector9 : BusSelector  OutputSignals=Driveline.EngSpd,Driveline.EMSpd,Driveline.Gear
  Bus to Vector : BusToVector
  Bus to Vector1 : BusToVector
  Bus to Vector2 : BusToVector
  Ground1 : Ground
  Max : MinMax  Function=max  Inputs=2
  Multi-Track XY Plotter : vehdynlibviscommon/Multi-Track XY Plotter  numTrack=Single track  extRef=on  extStats=on  extTireF=on  a=1.5  b=1.5  w=0  figBorder=10  bufferSize=1024  velNorm=5  tireFNorm=1000  pltDT=.1
      settings: LibrarySourceBlock=vehdynlibviscommon/Vehicle XY Plot Configuration
  Mux : Mux  Inputs=3
  Mux{1..4} (4 alike) : Mux  Inputs=2
  Unary Minus : UnaryMinus
  wires:
  Bus Selector7/1 -> Bus to Vector1/1
  Ground1/1 -> Mux/3
  Mux2/1 -> Unary Minus/1
  Bus to Vector1/1 -> Multi-Track XY Plotter/3
  Mux1/1 -> Multi-Track XY Plotter/7
  Bus Selector1/1 -> Bus to Vector2/1
  Bus Element In1/1 -> Mux/2
  Mux4/1 -> Multi-Track XY Plotter/6
  Bus Element In3/1 -> Mux/1
  Mux/1 -> Multi-Track XY Plotter/5
  Bus to Vector/1 -> Multi-Track XY Plotter/1
  Bus Selector6/1 -> Bus to Vector/1
  Bus to Vector2/1 -> Multi-Track XY Plotter/2
  Bus Selector5/1 -> Mux3/1  "<thetasteer>"
  Mux3/1 -> Multi-Track XY Plotter/4
  Bus Selector5/2 -> Mux3/2  "<Alpha>"
  Bus Selector10/1 -> Mux1/1  "<Fx>"
  Bus Selector10/2 -> Mux1/2  "<Fx>"
  Bus Selector10/3 -> Mux2/1  "<Fy>"
  Bus Selector10/4 -> Mux2/2  "<Fy>"
  Unary Minus/1 -> Multi-Track XY Plotter/8
  Bus Selector9/3 -> Mux4/2  "<Gear>"
  Bus Selector9/1 -> Max/1  "<EngSpd>"
  Bus Selector9/2 -> Max/2  "<EMSpd>"
  Max/1 -> Mux4/1
  Bus Element In2/1 -> Bus Selector9/1, Bus Selector10/1, Bus Selector5/1, Bus Selector7/1, Bus Selector1/1, Bus Selector6/1  "VehFdbk"

== system SiemensBike/Environment/Friction/Varying Friction/Road Track Friction ==
  XWhl : Inport
  YWhl : Inport  Port=2
  Cg : Inport  Port=3
  2D Lookup Tbl for Scaling Fctr (Lambda) : Subsystem  TreatAsAtomicUnit=on
      mask init:
      | [~]=vehdynicon('vehdynblk',gcb);
  Bus Selector : BusSelector  OutputSignals=X,Y
  Cnst Lambda : Constant  Value=ones(2,1).*lambda_g
  Constant1 : Constant  Value=SplitLambdaTrck
  Creating Inertial Frm Bpt : Subsystem
  En at t = 0 : Subsystem
  "Lambda (t = 0) " : Memory  InitialCondition=ones(2,1).*lambda_g  InheritSampleTime=on
  Switch : Switch  Criteria=u2 > Threshold  ZeroCross=off  SaturateOnIntegerOverflow=off  InputSameDT=off
  FricCoeffLambda : Outport
  wires:
  YWhl/1 -> 2D Lookup Tbl for Scaling Fctr (Lambda)/2(YWhl)
  XWhl/1 -> 2D Lookup Tbl for Scaling Fctr (Lambda)/1(XWhl)
  2D Lookup Tbl for Scaling Fctr (Lambda)/1(Lambda for each whl) -> Switch/1
  "Lambda (t = 0) "/1 -> FricCoeffLambda/1
  Switch/1 -> "Lambda (t = 0) "/1
  Cnst Lambda/1 -> Switch/3
  Constant1/1 -> Switch/2
  Cg/1 -> Bus Selector/1
  Creating Inertial Frm Bpt/1(XBpt) -> 2D Lookup Tbl for Scaling Fctr (Lambda)/3(XBpt)
  Creating Inertial Frm Bpt/2(YBpt) -> 2D Lookup Tbl for Scaling Fctr (Lambda)/4(YBpt)
  Bus Selector/1 -> Creating Inertial Frm Bpt/1(XCg)  "<X>"
  Bus Selector/2 -> Creating Inertial Frm Bpt/2(YCg)  "<Y>"
  En at t = 0/1(Out1) -> Creating Inertial Frm Bpt/Enable

== system SiemensBike/Environment/Friction/Varying Friction/Wheel Coordinates ==
  FrntAxlX : Inport
  RearAxlX : Inport  Port=2
  FrntAxlY : Inport  Port=3
  RearAxlY : Inport  Port=4
  Matrix Concatenate : Concatenate  Mode=Multidimensional array
  Matrix Concatenate1 : Concatenate  Mode=Multidimensional array
  XWhl : Outport
  YWhl : Outport  Port=2
  wires:
  Matrix Concatenate/1 -> XWhl/1
  FrntAxlX/1 -> Matrix Concatenate/1
  Matrix Concatenate1/1 -> YWhl/1
  FrntAxlY/1 -> Matrix Concatenate1/1
  RearAxlY/1 -> Matrix Concatenate1/2
  RearAxlX/1 -> Matrix Concatenate/2

== system SiemensBike/Environment/Ground Feedback/3D Engine/3D Engine Source ==
  WheelFdbk : Inport
  Multiple Points : Subsystem  VariantControl=terrType==2
  Single Point : Subsystem  VariantControl=terrType ==1
  z : Outport
  DCM : Outport  Port=2

== system SiemensBike/Motorcycle Vehicle/Hand Levers and Pedals/Hand Levers and Pedals/Brake Pedal ==
  DecelCmd : Inport
  Dead Zone1 : DeadZone  LowerValue=0  UpperValue=.01  ZeroCross=off
  DecelFdbk : Outport
  wires:
  Dead Zone1/1 -> DecelFdbk/1
  DecelCmd/1 -> Dead Zone1/1

== system SiemensBike/Motorcycle Vehicle/Transmission, Driveline and Brakes/Transmission and Driveline/Driveline ==
  FCpR : Inport
  ThetaFrm : Inport  Port=2
  ThetaArmR : Inport  Port=3
  MBrkR : Inport  Port=4
  AngAWhlR : Inport  Port=5
  DrvSprktTrq : Inport  Port=6
  Chain_Drive : Subsystem  VariantControl=Chain_Drive  ReferencedSubsystem=Chain_Drive
  No_Chain_Drive : Subsystem  VariantControl=No_Chain_Drive  ReferencedSubsystem=No_Chain_Drive
  Info : Outport
  DrvSprktSpd : Outport  Port=2

== system SiemensBike/Motorcycle Vehicle/Transmission, Driveline and Brakes/Transmission and Driveline/Transmission ==
  EngTrq : Inport
  GearCmd : Inport  Port=2
  EMTrq : Inport  Port=3
  DrvSprktSpd : Inport  Port=4
  ConventionalMotorcycle : Subsystem  VariantControl=ConventionalMotorcycle  ReferencedSubsystem=ConventionalMotorcycle
  ElectricMotorcycle : Subsystem  VariantControl=ElectricMotorcycle  ReferencedSubsystem=ElectricMotorcycle
  EngSpd : Outport
  Gear : Outport  Port=2
  EMSpd : Outport  Port=3
  DrvSprktTrq : Outport  Port=4

== system SiemensBike/Environment/Friction/Varying Friction/Road Track Friction/2D Lookup Tbl for Scaling Fctr (Lambda) ==
  XWhl : Inport  Partition=on  PartitionDimension=1  PartitionWidth=1  PartitionOffset=0
  YWhl : Inport  Port=2  Partition=on  PartitionDimension=1  PartitionWidth=1  PartitionOffset=0
  XBpt : Inport  Port=3
  YBpt : Inport  Port=4
  2-D Lookup Table : Lookup_n-D  BreakpointsForDimension1Source=Input port  BreakpointsForDimension1=xbr  BreakpointsForDimension2Source=Input port  BreakpointsForDimension2=ybr  Table=mutable  ExtrapMethod=Clip  InternalRulePriority=Speed  RndMeth=Simplest
      settings: InputPortMap=u0,u1,p5,p7
  For Each : ForEach  DisableCoverage=on
  Lambda for each whl : Outport  ConcatenationDimension=1
  wires:
  XWhl/1 -> 2-D Lookup Table/1
  YWhl/1 -> 2-D Lookup Table/2
  2-D Lookup Table/1 -> Lambda for each whl/1
  XBpt/1 -> 2-D Lookup Table/3
  YBpt/1 -> 2-D Lookup Table/4

== system SiemensBike/Environment/Friction/Varying Friction/Road Track Friction/Creating Inertial Frm Bpt ==
  XCg : Inport
  YCg : Inport  Port=2
  Enable : EnablePort
  Add : Sum
  Add1 : Sum
  Constant1 : Constant  Value=ybr
  Constant3 : Constant  Value=xbr
  XBpt : Outport
  YBpt : Outport  Port=2
  wires:
  Add/1 -> XBpt/1
  Constant1/1 -> Add1/1
  Add1/1 -> YBpt/1
  Constant3/1 -> Add/2
  YCg/1 -> Add1/2
  XCg/1 -> Add/1

== system SiemensBike/Environment/Friction/Varying Friction/Road Track Friction/En at t = 0 ==
  Clock1 : Clock
  Compare To Zero : simulink/Logic and Bit Operations/Compare To Zero  relop===  OutDataTypeStr=boolean
  Constant : Constant
  Constant2 : Constant  Value=0
  Switch1 : Switch  Criteria=u2 > Threshold  SaturateOnIntegerOverflow=off  InputSameDT=off
  Out1 : Outport
  wires:
  Clock1/1 -> Compare To Zero/1
  Constant2/1 -> Switch1/3
  Constant/1 -> Switch1/1
  Switch1/1 -> Out1/1
  Compare To Zero/1 -> Switch1/2

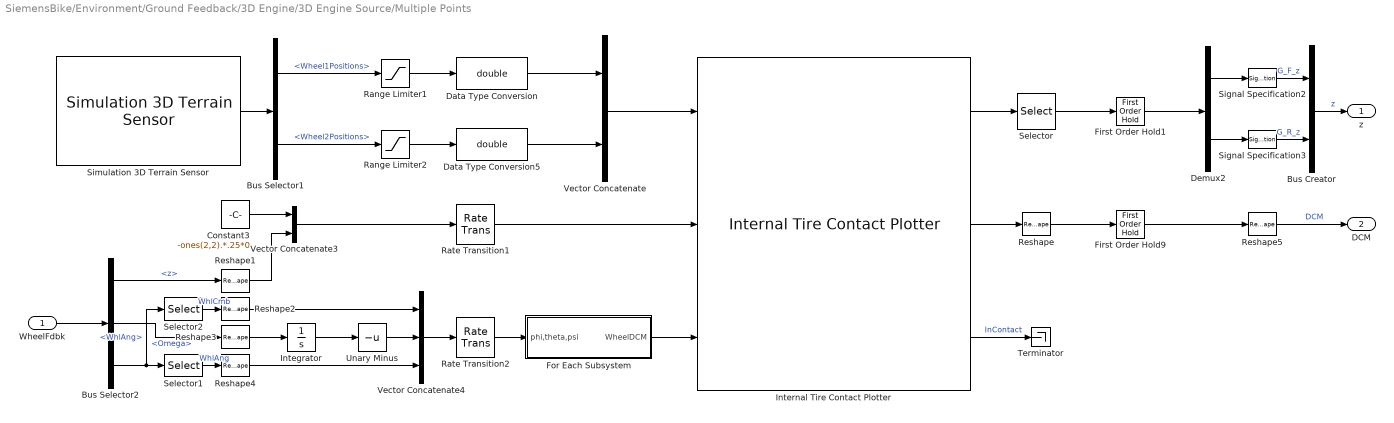
== system SiemensBike/Environment/Ground Feedback/3D Engine/3D Engine Source/Multiple Points ==
  WheelFdbk : Inport
  Bus Creator : BusCreator  Inputs=2
  Bus Selector1 : BusSelector  OutputSignals=Wheel1Positions,Wheel2Positions
  Bus Selector2 : BusSelector  OutputSignals=z,Omega,WhlAng
  Constant3 : Constant  Value=-ones(2,2).*.25*0
  Data Type Conversion : DataTypeConversion  OutDataTypeStr=double  SaturateOnIntegerOverflow=off  RndMeth=Floor
  Data Type Conversion5 : DataTypeConversion  OutDataTypeStr=double  SaturateOnIntegerOverflow=off  RndMeth=Floor
  Demux2 : Demux  Outputs=2
  First Order Hold1 : FirstOrderHold  OutputAlgorithm=Fast (Minimize Error)  ErrorTolerance=.001
  First Order Hold9 : FirstOrderHold  InitialOutput=reshape(repmat(eye(3),1,1,2),[],1)  OutputAlgorithm=Fast (Minimize Error)  ErrorTolerance=.001
  For Each Subsystem : Subsystem  TreatAsAtomicUnit=on
  Integrator : Integrator  WrapState=on  ZeroCross=off
  Internal Tire Contact Plotter : vehdynlibviscommon/Internal Tire Contact Plotter  dispFig=off  numAxles=2  numWheelsPerAxle=1  wheelRad=.33  wheelWidth=.235  rayOrigins=[0.5 -0.5 0;0.4 -0.5 0;0.3 -0.5 0;0.19999999999999996 -0.5 0;0.099999999999999978 -0.5 0;0 -0.5 0;-0.099999999999999978 -0.5 0;-0.19999999999999996 -0.5 0;-0.3 -0.5 0;-0.4 -0.5 0;-0.5 -0.5 0;0.5 -0.4 0;0.4 -0.4 0;0.3 -0.4 0;0.19999999999999996 -0.4 0;0.099999999999999978 -0.4 0;0 -0.4 0;-0.099999999999999978 -0.4 0;-0.19999999999999996 -0.4 0;-0.3 -0.4 0;-0.4 -0.4 0;-0.5 -0.4 0;0.5 -0.3 0;0.4 -0.3 0;0.3 -0.3 0;0.19999999999999996 -0.3 0;0.099999999999999978 -0.3 0;0 -0.3 0;-0.099999999999999978 -0.3 0;-0.19999999999999996 -0.3 0;-0.3 -0.3 0;-0.4 -0.3 0;-0.5 -0.3 0;0.5 -0.19999999999999996 0;0.4 -0.19999999999999996 0;0.3 -0.19999999999999996 0;0.19999999999999996 -0.19999999999999996 0;0.099999999999999978 -0.19999999999999996 0;0 -0.19999999999999996 0;-0.099999999999999978 -0.19999999999999996 0;-0.19999999999999996 -0.19999999999999996 0;-0.3 -0.19999999999999996 0;-0.4 -0.19999999999999996 0;-0.5 -0.19999999999999996 0;0.5 -0.099999999999999978 0;0.4 -0.099999999999999978 0;0.3 -0.099999999999999978 0;0.19999999999999996 -0.099999999999999978 0;0.099999999999999978 -0.099999999999999978 0;0 -0.099999999999999978 0;-0.099999999999999978 -0.099999999999999978 0;-0.19999999999999996 -0.099999999999999978 0;-0.3 -0.099999999999999978 0;-0.4 -0.099999999999999978 0;-0.5 -0.099999999999999978 0;0.5 0 0;0.4 0 0;0.3 0 0;0.19999999999999996 0 0;0.099999999999999978 0 0;0 0 0;-0.099999999999999978 0 0;-0.19999999999999996 0 0;-0.3 0 0;-0.4 0 0;-0.5 0 0;0.5 0.099999999999999978 0;0.4 0.099999999999999978 0;0.3 0.099999999999999978 0;0.19999999999999996 0.099999999999999978 0;0.099999999999999978 0.099999999999999978 0;0 0.099999999999999978 0;-0.099999999999999978 0.099999999999999978 0;-0.19999999999999996 0.099999999999999978 0;-0.3 0.099999999999999978 0;-0.4 0.099999999999999978 0;-0.5 0.099999999999999978 0;0.5 0.19999999999999996 0;0.4 0.19999999999999996 0;0.3 0.19999999999999996 0;0.19999999999999996 0.19999999999999996 0;0.099999999999999978 0.19999999999999996 0;0 0.19999999999999996 0;-0.099999999999999978 0.19999999999999996 0;-0.19999999999999996 0.19999999999999996 0;-0.3 0.19999999999999996 0;-0.4 0.19999999999999996 0;-0.5 0.19999999999999996 0;0.5 0.3 0;0.4 0.3 0;0.3 0.3 0;0.19999999999999996 0.3 0;0.099999999999999978 0.3 0;0 0.3 0;-0.099999999999999978 0.3 0;-0.19999999999999996 0.3 0;-0.3 0.3 0;-0.4 0.3 0;-0.5 0.3 0;0.5 0.4 0;0.4 0.4 0;0.3 0.4 0;0.19999999999999996 0.4 0;0.099999999999999978 0.4 0;0 0.4 0;-0.099999999999999978 0.4 0;-0.19999999999999996 0.4 0;-0.3 0.4 0;-0.4 0.4 0;-0.5 0.4 0;0.5 0.5 0;0.4 0.5 0;0.3 0.5 0;0.19999999999999996 0.5 0;0.099999999999999978 0.5 0;0 0.5 0;-0.099999999999999978 0.5 0;-0.19999999999999996 0.5 0;-0.3 0.5 0;-0.4 0.5 0;-0.5 0.5 0]
  Range Limiter1 : Saturate  UpperLimit=1e3  LowerLimit=-1e3  ZeroCross=off
  Range Limiter2 : Saturate  UpperLimit=1e3  LowerLimit=-1e3  ZeroCross=off
  Rate Transition1 : RateTransition  Integrity=off  Deterministic=off  OutPortSampleTime=.01
  Rate Transition2 : RateTransition  Integrity=off  Deterministic=off  OutPortSampleTime=.01
  Reshape : Reshape  OutputDimensionality=Column vector (2-D)
  Reshape1 : Reshape  OutputDimensionality=Column vector (2-D)
  Reshape2 : Reshape  OutputDimensionality=Row vector (2-D)
  Reshape3 : Reshape  OutputDimensionality=Row vector (2-D)
  Reshape4 : Reshape  OutputDimensionality=Row vector (2-D)
  Reshape5 : Reshape  OutputDimensionality=Customize  OutputDimensions=[3,3,2]
  Selector : Selector  NumberOfDimensions=2  InputPortWidth=3  IndexOptions=Select all,Index vector (dialog)  Indices=[1 3],3  OutputSizes=1,1
  Selector1 : Selector  NumberOfDimensions=2  InputPortWidth=3  IndexOptions=Index vector (dialog),Select all  Indices=[3],1  OutputSizes=1,1
  Selector2 : Selector  NumberOfDimensions=2  InputPortWidth=3  IndexOptions=Index vector (dialog),Select all  Indices=[1],1  OutputSizes=1,1
  Signal Specification2 : SignalSpecification  Unit=m
  Signal Specification3 : SignalSpecification  Unit=m
  Simulation 3D Terrain Sensor : sim3dgroundtruthsensorlib/Simulation 3D Terrain Sensor  Priority=1  vehTagList={'Scene Origin';'SimulinkVehicle1'}  sensorTag=Sim3dSensor�  sensorId=1  sensorName=Sim3dSensor�  vehTag=SimulinkVehicle1  CoordinateSystem=Default  tmountOffset=[0, 0, 0]  rmountOffset=[0,0,0,]  RayOrigins=[0.5 -0.5 0;0.4 -0.5 0;0.3 -0.5 0;0.19999999999999996 -0.5 0;0.099999999999999978 -0.5 0;0 -0.5 0;-0.099999999999999978 -0.5 0;-0.19999999999999996 -0.5 0;-0.3 -0.5 0;-0.4 -0.5 0;-0.5 -0.5 0;0.5 -0.4 0;0.4 -0.4 0;0.3 -0.4 0;0.19999999999999996 -0.4 0;0.099999999999999978 -0.4 0;0 -0.4 0;-0.099999999999999978 -0.4 0;-0.19999999999999996 -0.4 0;-0.3 -0.4 0;-0.4 -0.4 0;-0.5 -0.4 0;0.5 -0.3 0;0.4 -0.3 0;0.3 -0.3 0;0.19999999999999996 -0.3 0;0.099999999999999978 -0.3 0;0 -0.3 0;-0.099999999999999978 -0.3 0;-0.19999999999999996 -0.3 0;-0.3 -0.3 0;-0.4 -0.3 0;-0.5 -0.3 0;0.5 -0.19999999999999996 0;0.4 -0.19999999999999996 0;0.3 -0.19999999999999996 0;0.19999999999999996 -0.19999999999999996 0;0.099999999999999978 -0.19999999999999996 0;0 -0.19999999999999996 0;-0.099999999999999978 -0.19999999999999996 0;-0.19999999999999996 -0.19999999999999996 0;-0.3 -0.19999999999999996 0;-0.4 -0.19999999999999996 0;-0.5 -0.19999999999999996 0;0.5 -0.099999999999999978 0;0.4 -0.099999999999999978 0;0.3 -0.099999999999999978 0;0.19999999999999996 -0.099999999999999978 0;0.099999999999999978 -0.099999999999999978 0;0 -0.099999999999999978 0;-0.099999999999999978 -0.099999999999999978 0;-0.19999999999999996 -0.099999999999999978 0;-0.3 -0.099999999999999978 0;-0.4 -0.099999999999999978 0;-0.5 -0.099999999999999978 0;0.5 0 0;0.4 0 0;0.3 0 0;0.19999999999999996 0 0;0.099999999999999978 0 0;0 0 0;-0.099999999999999978 0 0;-0.19999999999999996 0 0;-0.3 0 0;-0.4 0 0;-0.5 0 0;0.5 0.099999999999999978 0;0.4 0.099999999999999978 0;0.3 0.099999999999999978 0;0.19999999999999996 0.099999999999999978 0;0.099999999999999978 0.099999999999999978 0;0 0.099999999999999978 0;-0.099999999999999978 0.099999999999999978 0;-0.19999999999999996 0.099999999999999978 0;-0.3 0.099999999999999978 0;-0.4 0.099999999999999978 0;-0.5 0.099999999999999978 0;0.5 0.19999999999999996 0;0.4 0.19999999999999996 0;0.3 0.19999999999999996 0;0.19999999999999996 0.19999999999999996 0;0.099999999999999978 0.19999999999999996 0;0 0.19999999999999996 0;-0.099999999999999978 0.19999999999999996 0;-0.19999999999999996 0.19999999999999996 0;-0.3 0.19999999999999996 0;-0.4 0.19999999999999996 0;-0.5 0.19999999999999996 0;0.5 0.3 0;0.4 0.3 0;0.3 0.3 0;0.19999999999999996 0.3 0;0.099999999999999978 0.3 0;0 0.3 0;-0.099999999999999978 0.3 0;-0.19999999999999996 0.3 0;-0.3 0.3 0;-0.4 0.3 0;-0.5 0.3 0;0.5 0.4 0;0.4 0.4 0;0.3 0.4 0;0.19999999999999996 0.4 0;0.099999999999999978 0.4 0;0 0.4 0;-0.099999999999999978 0.4 0;-0.19999999999999996 0.4 0;-0.3 0.4 0;-0.4 0.4 0;-0.5 0.4 0;0.5 0.5 0;0.4 0.5 0;0.3 0.5 0;0.19999999999999996 0.5 0;0.099999999999999978 0.5 0;0 0.5 0;-0.099999999999999978 0.5 0;-0.19999999999999996 0.5 0;-0.3 0.5 0;-0.4 0.5 0;-0.5 0.5 0]  RayDirections=[0 0 -1;0 0 -1;0 0 -1;0 0 -1;0 0 -1;0 0 -1;0 0 -1;0 0 -1;0 0 -1;0 0 -1;0 0 -1;0 0 -1;0 0 -1;0 0 -1;0 0 -1;0 0 -1;0 0 -1;0 0 -1;0 0 -1;0 0 -1;0 0 -1;0 0 -1;0 0 -1;0 0 -1;0 0 -1;0 0 -1;0 0 -1;0 0 -1;0 0 -1;0 0 -1;0 0 -1;0 0 -1;0 0 -1;0 0 -1;0 0 -1;0 0 -1;0 0 -1;0 0 -1;0 0 -1;0 0 -1;0 0 -1;0 0 -1;0 0 -1;0 0 -1;0 0 -1;0 0 -1;0 0 -1;0 0 -1;0 0 -1;0 0 -1;0 0 -1;0 0 -1;0 0 -1;0 0 -1;0 0 -1;0 0 -1;0 0 -1;0 0 -1;0 0 -1;0 0 -1;0 0 -1;0 0 -1;0 0 -1;0 0 -1;0 0 -1;0 0 -1;0 0 -1;0 0 -1;0 0 -1;0 0 -1;0 0 -1;0 0 -1;0 0 -1;0 0 -1;0 0 -1;0 0 -1;0 0 -1;0 0 -1;0 0 -1;0 0 -1;0 0 -1;0 0 -1;0 0 -1;0 0 -1;0 0 -1;0 0 -1;0 0 -1;0 0 -1;0 0 -1;0 0 -1;0 0 -1;0 0 -1;0 0 -1;0 0 -1;0 0 -1;0 0 -1;0 0 -1;0 0 -1;0 0 -1;0 0 -1;0 0 -1;0 0 -1;0 0 -1;0 0 -1;0 0 -1;0 0 -1;0 0 -1;0 0 -1;0 0 -1;0 0 -1;0 0 -1;0 0 -1;0 0 -1;0 0 -1;0 0 -1;0 0 -1;0 0 -1;0 0 -1;0 0 -1;0 0 -1;0 0 -1]  RayLengths=[20;20;20;20;20;20;20;20;20;20;20;20;20;20;20;20;20;20;20;20;20;20;20;20;20;20;20;20;20;20;20;20;20;20;20;20;20;20;20;20;20;20;20;20;20;20;20;20;20;20;20;20;20;20;20;20;20;20;20;20;20;20;20;20;20;20;20;20;20;20;20;20;20;20;20;20;20;20;20;20;20;20;20;20;20;20;20;20;20;20;20;20;20;20;20;20;20;20;20;20;20;20;20;20;20;20;20;20;20;20;20;20;20;20;20;20;20;20;20;20;20]  NumberOfWheels=2  VisualizeTraceLines=off  SampleTime=-1  aMode=2  ID=1
  Terminator : Terminator
  Unary Minus : UnaryMinus
  Vector Concatenate : Concatenate  Mode=Multidimensional array  ConcatenateDimension=3
  Vector Concatenate3 : Concatenate  Mode=Multidimensional array  ConcatenateDimension=2
  Vector Concatenate4 : Concatenate  NumInputs=3  Mode=Multidimensional array
  z : Outport
  DCM : Outport  Port=2
  wires:
  Selector2/1 -> Reshape2/1  "WhlCmb"
  Selector1/1 -> Reshape4/1  "WhlAng"
  First Order Hold1/1 -> Demux2/1
  Reshape/1 -> First Order Hold9/1
  First Order Hold9/1 -> Reshape5/1
  Rate Transition1/1 -> Internal Tire Contact Plotter/2
  Unary Minus/1 -> Vector Concatenate4/2
  Reshape2/1 -> Vector Concatenate4/1
  Constant3/1 -> Vector Concatenate3/1
  Bus Selector2/3 -> Selector1/1, Selector2/1  "<WhlAng>"
  Bus Selector2/1 -> Reshape1/1  "<z>"
  WheelFdbk/1 -> Bus Selector2/1
  Reshape1/1 -> Vector Concatenate3/2
  Rate Transition2/1 -> For Each Subsystem/1(phi,theta,psi)
  Reshape4/1 -> Vector Concatenate4/3
  Vector Concatenate4/1 -> Rate Transition2/1
  Reshape3/1 -> Integrator/1
  For Each Subsystem/1(WheelDCM) -> Internal Tire Contact Plotter/3
  Vector Concatenate3/1 -> Rate Transition1/1
  Bus Selector2/2 -> Reshape3/1  "<Omega>"
  Integrator/1 -> Unary Minus/1
  Internal Tire Contact Plotter/2 -> Reshape/1
  Reshape5/1 -> DCM/1  "DCM"
  Range Limiter1/1 -> Data Type Conversion/1
  Simulation 3D Terrain Sensor/1 -> Bus Selector1/1
  Demux2/1 -> Signal Specification2/1
  Bus Selector1/2 -> Range Limiter2/1  "<Wheel2Positions>"
  Signal Specification3/1 -> Bus Creator/2  "G_R_z"
  Signal Specification2/1 -> Bus Creator/1  "G_F_z"
  Bus Creator/1 -> z/1  "z"
  Bus Selector1/1 -> Range Limiter1/1  "<Wheel1Positions>"
  Vector Concatenate/1 -> Internal Tire Contact Plotter/1
  Internal Tire Contact Plotter/3 -> Terminator/1  "InContact"
  Internal Tire Contact Plotter/1 -> Selector/1
  Data Type Conversion5/1 -> Vector Concatenate/2
  Data Type Conversion/1 -> Vector Concatenate/1
  Demux2/2 -> Signal Specification3/1
  Selector/1 -> First Order Hold1/1
  Range Limiter2/1 -> Data Type Conversion5/1
